simulink model "FilterBLT"  (R2020b)
settings: Solver=VariableStepAuto  StartTime=0.0  StopTime=0.05  MaxStep=0.00001  RelTol=1e-3
settings Model: Creator=BIDITA PAUL  LastModifiedBy=BIDITA PAUL

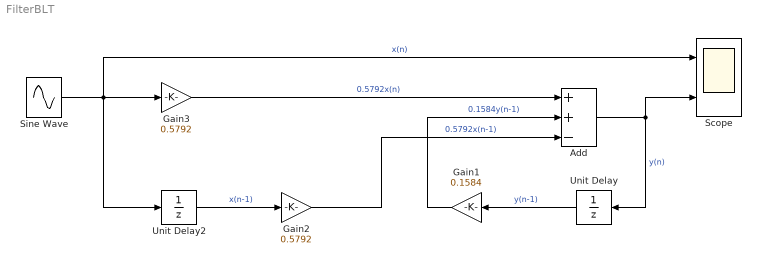
== system FilterBLT ==
  Add : Sum  Inputs=++-
  Gain1 : Gain  Gain=0.1584
  Gain2 : Gain  Gain=0.5792
  Gain3 : Gain  Gain=0.5792
  Scope : Scope  NumInputPorts=2
  Sine Wave : Sin  Frequency=2*pi*1000  SampleTime=0
  Unit Delay : UnitDelay  SampleTime=-1  HasFrameUpgradeWarning=on
  Unit Delay2 : UnitDelay  SampleTime=-1  HasFrameUpgradeWarning=on
  wires:
  Add/1 -> Unit Delay/1, Scope/2  "y(n)"
  Sine Wave/1 -> Scope/1, Unit Delay2/1, Gain3/1  "x(n)"
  Unit Delay2/1 -> Gain2/1  "x(n-1)"
  Unit Delay/1 -> Gain1/1  "y(n-1)"
  Gain2/1 -> Add/3  "0.5792x(n-1)"
  Gain3/1 -> Add/1  "0.5792x(n)"
  Gain1/1 -> Add/2  "0.1584y(n-1)"
